simulink model "ElevResp2"  (Simulink 6.5)
settings: Solver=ode45  StartTime=0.0  StopTime=100  RelTol=1e-3
settings Model: Creator=douglast  LastModifiedBy=douglast  ExtModeAutoUpdateStatusClock=off

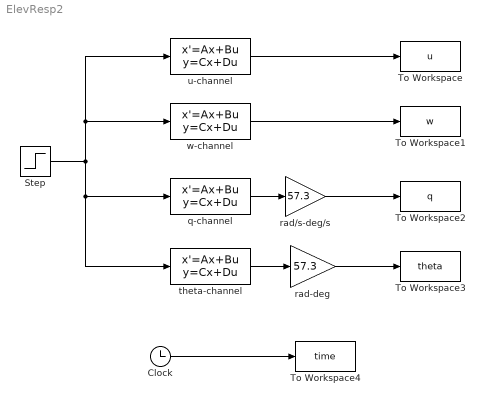
== system ElevResp2 ==
  Clock : Clock
      settings: Decimation=10
  Step : Step  Time=0  After=0.01745  SampleTime=0
  To Workspace : ToWorkspace  VariableName=u  SampleTime=-1  SaveFormat=Array
  To Workspace1 : ToWorkspace  VariableName=w  SampleTime=-1  SaveFormat=Array
  To Workspace2 : ToWorkspace  VariableName=q  SampleTime=-1  SaveFormat=Array
  To Workspace3 : ToWorkspace  VariableName=theta  SampleTime=-1  SaveFormat=Array
  To Workspace4 : ToWorkspace  VariableName=time  SampleTime=-1  SaveFormat=Array
  q-channel : StateSpace  A=[-0.06728 0.02323 0.0 -9.81; -0.396 -1.729 50.0 0.0; 0.0078 -0.2431 -3.192 0.0;0 0 1 0]  B=[0;-17.01;-44.37;0]  C=[0 0 1 0]  D=0
  rad-deg : Gain  Gain=57.3
  rad/s-deg/s : Gain  Gain=57.3
  theta-channel : StateSpace  A=[-0.06728 0.02323 0.0 -9.81; -0.396 -1.729 50.0 0.0; 0.0078 -0.2431 -3.192 0.0;0 0 1 0]  B=[0;-17.01;-44.37;0]  C=[0 0 0 1]  D=0
  u-channel : StateSpace  A=[-0.06728 0.02323 0.0 -9.81; -0.396 -1.729 50.0 0.0; 0.0078 -0.2431 -3.192 0.0;0 0 1 0]  B=[0;-17.01;-44.37;0]  C=[1 0 0 0]  D=0
  w-channel : StateSpace  A=[-0.06728 0.02323 0.0 -9.81; -0.396 -1.729 50.0 0.0; 0.0078 -0.2431 -3.192 0.0;0 0 1 0]  B=[0;-17.01;-44.37;0]  C=[0 1 0 0]  D=0
  wires:
  Step/1 -> u-channel/1, w-channel/1, theta-channel/1, q-channel/1
  q-channel/1 -> rad/s-deg/s/1
  theta-channel/1 -> rad-deg/1
  u-channel/1 -> To Workspace/1
  w-channel/1 -> To Workspace1/1
  rad/s-deg/s/1 -> To Workspace2/1
  rad-deg/1 -> To Workspace3/1
  Clock/1 -> To Workspace4/1
